simulink model "d_analog_ss"  (R2019b)
settings: Solver=VariableStepAuto  StartTime=0.0  StopTime=10.0  RelTol=1e-3
values from neighbouring files (symbols this model uses):
  K1 = 1 + 0.1*(2*rand()-1)    [diffcode.m]
  K2 = 1 + 0.1*(2*rand()-1)    [diffcode.m]
  Kd = 1/(exp(T0/Kda)-1)    [diffcode.m]
  Kda = T1    (= 0.1)    [diffcode.m]
  Kp = Kpa    (= 1)    [diffcode.m]
  Kpa = 1/(2*Tu*K1*K2)    [diffcode.m]
  st = 1    [diffcode.m]
  T0 = 0.1    [diffcode.m]
  T1 = 1 + 0.1*(2*rand()-1)    [diffcode.m]
  Tur = T0/2    (= 0.05)    [diffcode.m]
settings Model: Creator=bedla  LastModifiedBy=bedla
settings DataIOCC: ReturnWorkspaceOutputs=off

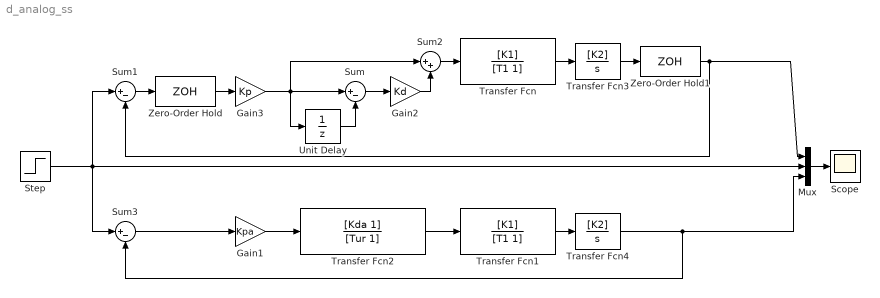
== system d_analog_ss ==
  Gain1 : Gain  Gain=Kpa
  Gain2 : Gain  Gain=Kd
  Gain3 : Gain  Gain=Kp
  Mux : Mux  Inputs=3
  Scope : Scope
  Step : Step  After=st  SampleTime=0
  Sum : Sum  Inputs=|+-
  Sum1 : Sum  Inputs=|+-
  Sum2 : Sum  Inputs=|++
  Sum3 : Sum  Inputs=|+-
  Transfer Fcn : TransferFcn  Numerator=[K1]  Denominator=[T1 1]
  Transfer Fcn1 : TransferFcn  Numerator=[K1]  Denominator=[T1 1]
  Transfer Fcn2 : TransferFcn  Numerator=[Kda 1]  Denominator=[Tur 1]
  Transfer Fcn3 : TransferFcn  Numerator=[K2]  Denominator=[1 0]
  Transfer Fcn4 : TransferFcn  Numerator=[K2]  Denominator=[1 0]
  Unit Delay : UnitDelay  SampleTime=T0  HasFrameUpgradeWarning=on
  Zero-Order Hold : ZeroOrderHold  SampleTime=T0
  Zero-Order Hold1 : ZeroOrderHold  SampleTime=T0
  wires:
  Sum2/1 -> Transfer Fcn/1
  Transfer Fcn1/1 -> Transfer Fcn4/1
  Sum/1 -> Gain2/1
  Step/1 -> Sum3/1, Sum1/1, Mux/2
  Mux/1 -> Scope/1
  Zero-Order Hold/1 -> Gain3/1
  Transfer Fcn2/1 -> Transfer Fcn1/1
  Unit Delay/1 -> Sum/2
  Gain2/1 -> Sum2/2
  Zero-Order Hold1/1 -> Sum1/2, Mux/1
  Gain3/1 -> Sum2/1, Sum/1, Unit Delay/1
  Transfer Fcn/1 -> Transfer Fcn3/1
  Transfer Fcn3/1 -> Zero-Order Hold1/1
  Sum1/1 -> Zero-Order Hold/1
  Gain1/1 -> Transfer Fcn2/1
  Transfer Fcn4/1 -> Sum3/2, Mux/3
  Sum3/1 -> Gain1/1
